simulink library "HeatExchanger"  (R2018b)
settings: Solver=ode45  StartTime=0.0  StopTime=10.0  RelTol=1e-3  EnableMultiTasking=on
libraries: carnot x2
settings Model: Creator=lena.frank  LastModifiedBy=P41573
settings DataIOCC: LimitDataPoints=on  SaveFormat=Array  SignalLoggingSaveFormat=ModelDataLogs
settings OptimizationCC: ExpressionDepthLimit=2147483647  LifeSpan=inf
settings DebuggingCC: UnderspecifiedInitializationDetection=Classic  MergeDetectMultiDrivingBlocksExec=none  SolverPrmCheckMsg=warning  FcnCallInpInsideContextMsg=warning  StateNameClashWarn=warning  SFUnexpectedBacktrackingDiag=warning  SFNoUnconditionalDefaultTransitionDiag=warning  SFExecutionAtInitializationDiag=none
settings HardwareCC: ProdBitPerPointer=32  ProdBitPerSizeT=32  ProdBitPerPtrDiffT=32  ProdLargestAtomicFloat=None  ProdIntDivRoundTo=Undefined  ProdEndianess=Unspecified  ProdWordSize=32  ProdHWDeviceType=32-bit Generic
settings ModelReferenceCC: PropagateSignalLabelsOutOfModel=off
settings SFSimCC: SimUseLocalCustomCode=off
settings RTWCC: RTWUseLocalCustomCode=off
settings CodeAppCC: StateflowObjectComments=on
settings GRTTargetCC: TargetLangStandard=C89/C90 (ANSI)  GeneratePreprocessorConditionals=Disable all  CombineOutputUpdateFcns=off  GRTInterface=on
settings ConfigComp: CovMetricSettings=dw  CovHtmlReporting=on  CovSaveCumulativeToWorkspaceVar=on  CovSaveSingleToWorkspaceVar=on  CovExternalEMLEnable=off

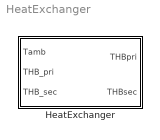
== system HeatExchanger ==
  HeatExchanger : Subsystem  mask(heat exchanger){flowtype=1, ua0=2000, uahot=[0.1 0], uacold=[0.1 0], ualoss=1, cap=2*4182, linh=20, quah=10, linc=20, quac=10, t0=20}
      mask prompts: flowtype "type of flow (0 = parallel, 0.5 = cross, 1 = counter)"; ua0 "constant heat transfer ua0 [W/K]"; uahot "[mdot_nom_pri [kg/s],  ua_exp_pri]"; uacold "[mdot_nom_sec [kg/s],  ua_exp_sec]"; ualoss "heat losses to ambient [W/K]"; cap "capacity [J/K]"; linh "Source: pressure drop linear in massflow [Pa*s/kg]"; quah "Source: pressure drop quadratic in massflow [Pa*s²/kg²]"; linc "Load: pressure drop linear in massflow [Pa*s/kg]"; quac "Load: pressure drop quadratic in massflow [Pa*s²/kg²]"; t0 "initial temperature [degree centigrade]"
      mask help:
      | Model of a heat exchanger using the NTU approach
      | The heat transfer is:
      | ua = ua0 * ( (mdot_pri/mdot_nom_pri)^ua_exp_pri
      |      + (mdot_sec/mdot_nom_sec)^ua_exp_sec )/2
      mask Help: web(fullfile(path_carnot('help'),'HeatExchanger.html'),'-helpbrowser')
      mask DialogControl ParameterTabVar0 Prompt: Thermal
      mask DialogControl ParameterTabVar01 Prompt: Hydraulic
      mask DialogControl ParameterTabVar012 Prompt: Calculation
      mask Display: plot(-10,20,115,100,[40,70,70,40,40],[40 40 70 70 40],[55 55 62 48 55 55],[25 40 55 55 70 85],[30 40],[55 55],[70 80],[55 55])

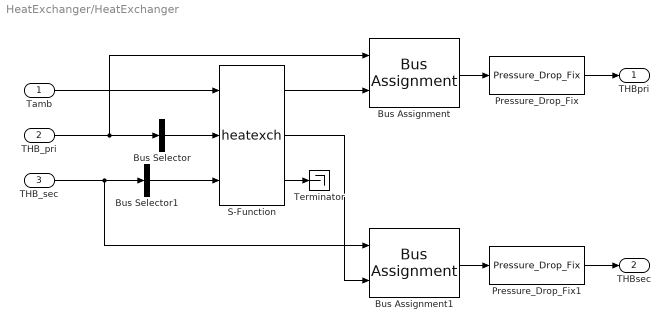
== system HeatExchanger/HeatExchanger ==
  Tamb : Inport
  THB_pri : Inport  Port=2
  THB_sec : Inport  Port=3
  Bus Assignment : BusAssignment  AssignedSignals=Temperature
  Bus Assignment1 : BusAssignment  AssignedSignals=Temperature
  Bus Selector : BusSelector  OutputSignals=Temperature,MassFlow,Pressure,FluidType,FluidMix  OutputAsBus=on
  Bus Selector1 : BusSelector  OutputSignals=Temperature,MassFlow,Pressure,FluidType,FluidMix  OutputAsBus=on
  Pressure_Drop_Fix : carnot/Basic/Pressure_Drop/Pressure_Drop_Fix  con=0  lin=linh  qua=quah
      settings: SourceProductName=Carnot
  Pressure_Drop_Fix1 : carnot/Basic/Pressure_Drop/Pressure_Drop_Fix  con=0  lin=linc  qua=quac
      settings: SourceProductName=Carnot
  S-Function : S-Function  FunctionName=heatexch  Parameters=flowtype, ua0, uahot(1), uahot(2), uacold(1), uacold(2), ualoss, cap, t0  SFunctionDeploymentMode=off  EnableBusSupport=off
  Terminator : Terminator
  THBpri : Outport
  THBsec : Outport  Port=2
  wires:
  Tamb/1 -> S-Function/1
  Bus Selector/1 -> S-Function/2
  S-Function/3 -> Terminator/1
  THB_pri/1 -> Bus Selector/1, Bus Assignment/1
  THB_sec/1 -> Bus Selector1/1, Bus Assignment1/1
  Bus Selector1/1 -> S-Function/3
  S-Function/1 -> Bus Assignment/2
  Bus Assignment/1 -> Pressure_Drop_Fix/1
  S-Function/2 -> Bus Assignment1/2
  Bus Assignment1/1 -> Pressure_Drop_Fix1/1
  Pressure_Drop_Fix/1 -> THBpri/1
  Pressure_Drop_Fix1/1 -> THBsec/1
